simulink model "switch_control"  (Simulink 7.6)
settings: Solver=FixedStepDiscrete  StartTime=0.0  StopTime=10.0  RelTol=1e-3
InitFcn:
  | %% DSPBuilder Start
  | alt_dspbuilder_update_model(bdroot)
  | %% DSPBuilder End
libraries: allblocks_alteradspbuilder2 x11, Stratix_III_DE3_260_alteradspbuilder2 x6
settings Model: Creator=akarapet  LastModifiedBy=akarapet
settings DataIOCC: SignalLoggingName=sigsOut
settings OptimizationCC: BlockReduction=off  BooleanDataType=off  InlineInvariantSignals=on  InitFltsAndDblsToZero=on
settings DebuggingCC: SaveWithParameterizedLinksMsg=none  SignalResolutionControl=TryResolveAllWithWarning  SolverPrmCheckMsg=none  MultiTaskDSMMsg=warning  MultiTaskCondExecSysMsg=none  StrictBusMsg=Warning
settings HardwareCC: TargetUnknown=on
settings RTWCC: IncludeERTFirstTime=on
settings GRTTargetCC: TargetFcnLib=ansi_tfl_tmw.mat

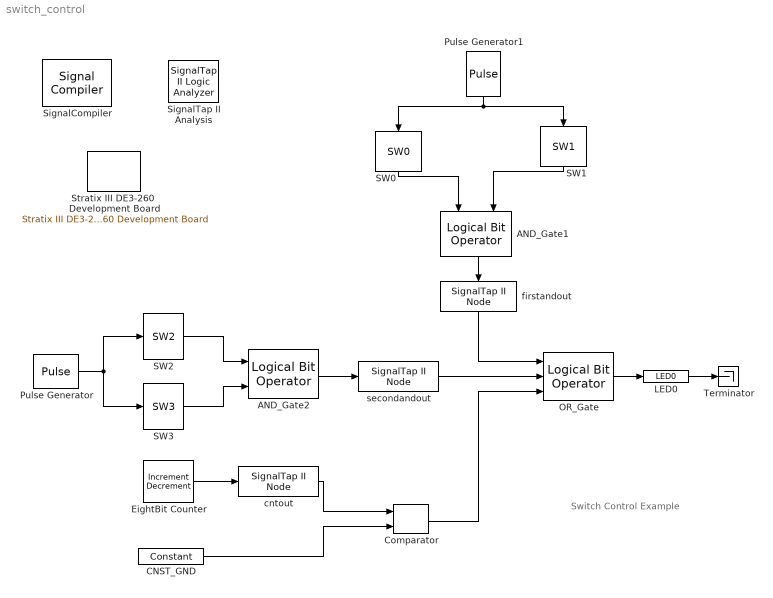
== system switch_control ==
  note: Switch Control Example
  AND_Gate1 : allblocks_alteradspbuilder2/Logical Bit Operator  LogicalOperator=AND  user_inputs=2  pipeline_display=0
  AND_Gate2 : allblocks_alteradspbuilder2/Logical Bit Operator  LogicalOperator=AND  user_inputs=2  pipeline_display=0
  CNST_GND : allblocks_alteradspbuilder2/Constant  mask_cst=0  BusType=Unsigned Integer  bwl=8  bwr=0  roundMode=Truncate  satMode=Wrap  SpecifyClock=off  allowFloatingPointOverride=on  logOutputs=off  logFile=/data/akarapet/qshell_linux64_test/p4/dsp_builder/dsp_builder2/Documentation/DesignExamples/Tutorials/SignalTap/professional/completed_walkthrough/tb_switch_control/switch%5Fcontrol_CNST%5FGND.fixedpointlog
  Comparator : allblocks_alteradspbuilder2/Comparator  direction=a == b  pipeline_display=0  allowFloatingPointOverride=on  logOutputs=off  logFile=/data/akarapet/qshell_linux64_test/p4/dsp_builder/dsp_builder2/Documentation/DesignExamples/Tutorials/SignalTap/professional/completed_walkthrough/tb_switch_control/switch%5Fcontrol_Comparator.fixedpointlog
  EightBit Counter : allblocks_alteradspbuilder2/Increment Decrement  BusType=Unsigned Integer  bwl=8  bwr=0  SpecifyClock=off  clr_value=0  direction=Increment  phase_selection=1  use_ena=off  use_sclr=off  pipeline_display=1
  LED0 : Stratix_III_DE3_260_alteradspbuilder2/LED0  iofile=/data/akarapet/qshell_linux64_test/p4/dsp_builder/dsp_builder2/Documentation/DesignExamples/Tutorials/SignalTap/professional/completed_walkthrough/tb_switch_control/switch%5Fcontrol_LED0.capture  externalType=Inferred  location=Pin_AD1
  OR_Gate : allblocks_alteradspbuilder2/Logical Bit Operator  LogicalOperator=OR  user_inputs=3  pipeline_display=0
  Pulse Generator : DiscretePulseGenerator  PulseType=Time based  PulseWidth=50
  Pulse Generator1 : DiscretePulseGenerator  PulseType=Time based  PulseWidth=50
  SW0 : Stratix_III_DE3_260_alteradspbuilder2/SW0  iofile=/data/akarapet/qshell_linux64_test/p4/dsp_builder/dsp_builder2/Documentation/DesignExamples/Tutorials/SignalTap/professional/completed_walkthrough/tb_switch_control/switch%5Fcontrol_SW0.salt  externalType=Inferred  SpecifyClock=off  location=Pin_W5
  SW1 : Stratix_III_DE3_260_alteradspbuilder2/SW1  iofile=/data/akarapet/qshell_linux64_test/p4/dsp_builder/dsp_builder2/Documentation/DesignExamples/Tutorials/SignalTap/professional/completed_walkthrough/tb_switch_control/switch%5Fcontrol_SW1.salt  externalType=Inferred  SpecifyClock=off  location=Pin_W6
  SW2 : Stratix_III_DE3_260_alteradspbuilder2/SW2  iofile=/data/akarapet/qshell_linux64_test/p4/dsp_builder/dsp_builder2/Documentation/DesignExamples/Tutorials/SignalTap/professional/completed_walkthrough/tb_switch_control/switch%5Fcontrol_SW2.salt  externalType=Inferred  SpecifyClock=off  location=Pin_W9
  SW3 : Stratix_III_DE3_260_alteradspbuilder2/SW3  iofile=/data/akarapet/qshell_linux64_test/p4/dsp_builder/dsp_builder2/Documentation/DesignExamples/Tutorials/SignalTap/professional/completed_walkthrough/tb_switch_control/switch%5Fcontrol_SW3.salt  externalType=Inferred  SpecifyClock=off  location=Pin_W11
  SignalCompiler : allblocks_alteradspbuilder2/Signal Compiler  DeviceFamily=Stratix III  DeviceName=EP3SE260F1152C2  EnableSignalTap=on  SignalTapDepth=128  UseBoardBlock=on  StpUseDefaultClock=on  StpClock=Clock  ExportDir=/data/akarapet/qshell_linux64_test/p4/dsp_builder/dsp_builder2/Documentation/DesignExamples/Tutorials/SignalTap
  SignalTap II Analysis : allblocks_alteradspbuilder2/SignalTap II Logic Analyzer
  Stratix III DE3-260  Development Board : Stratix_III_DE3_260_alteradspbuilder2/Stratix III DE3-260 Development Board  ClockPinIn=Pin_T33  GlobalResetPin=Pin_U31  device=EP3SE260F1152C2
  Terminator : Terminator
  cntout : allblocks_alteradspbuilder2/SignalTap II Node  id=0
  firstandout : allblocks_alteradspbuilder2/SignalTap II Node  id=1
  secondandout : allblocks_alteradspbuilder2/SignalTap II Node  id=2
  wires:
  SW2/1 -> AND_Gate2/1
  SW3/1 -> AND_Gate2/2
  EightBit Counter/1 -> cntout/1
  CNST_GND/1 -> Comparator/2
  AND_Gate2/1 -> secondandout/1
  Comparator/1 -> OR_Gate/3
  OR_Gate/1 -> LED0/1
  cntout/1 -> Comparator/1
  AND_Gate1/1 -> firstandout/1
  SW1/1 -> AND_Gate1/2
  SW0/1 -> AND_Gate1/1
  firstandout/1 -> OR_Gate/1
  secondandout/1 -> OR_Gate/2
  LED0/1 -> Terminator/1
  Pulse Generator/1 -> SW2/1, SW3/1
  Pulse Generator1/1 -> SW0/1, SW1/1
